simulink model "five_bar_model_with_gravity"  (R2018a)
settings: Solver=ode4  StartTime=0.0  StopTime=10  FixedStep=0.0001  RelTol=1e-3
values from neighbouring files (symbols this model uses):
  g = 9.80665    [ddyn5.m]    (also in idyn5.m = -9.80665; test_dynamics.m = -9.80665; test_model.m)
  q = [NaN; NaN; NaN; NaN; NaN]    [fkine5.m]    (also in ikine5.m = [q11;q12;q13;q21;q22])
  qa = [q11;q21]    [ikine5.m]    (also in model_parameters_v_1.m = ones(length(q_(1,:)),1) * 50; test_model.m = [q(1,:);q(4,:)])
  qda = Jinv * t0r    [ifirstkine5.m]    (also in test_model.m = [0.5; 0.5])
  t0r = J * qda    [ffirstkine5.m]    (also in test_dynamics.m = [0;0]; test_kinematics.m = [1;1]; test_model.m = p)
  t0rd = (J * qdda+ at)    [fsecondkine5.m]    (also in test_dynamics.m = [0;0]; test_kinematics.m = [-1;1]; test_model.m = p)
  x0 = p(1,1)    [model_parameters_v_1.m]    (also in test_model.m)
  y0 = p(2,1)    [model_parameters_v_1.m]    (also in test_model.m = p(1,2))
undefined symbols (not defined in the file or in its folder): X, Y, Z
libraries: sm_lib x25, nesl_utility x9, simulink x7, fl_lib x2
(part 2 of 2)

== matlab function five_bar_model_with_gravity/inverse first kinematics ==
  data: t0r input; qd output; p input double size=2; q input; qda output; qdu output; Ar output; B output; J output; Jinv output; Jt output; Jta output; Jtd output; Psit output
function [qd,qda,qdu,Ar,B,J,Jinv,Jt,Jta,Jtd,Psit] = ifirstkine5(t0r,p,q)
% This function implement the firs-order inverse kinematics model of a five bar robot
% @param t0r: twist end-effector vector 2X1
% @param p: end-effector coordinate vector 2X1
% @param q: joint positions vector 5x1
% @return qd: velocity joints vector 5x1
% @return qda: active velocity joints vector 2X1
% @return qdu: underactuated velocity joints vector 3X1
% @return Ar: matrix 2x2 relates the n dof independent coordinates of the platform twist 0 t r to the actuated joints q̇ a
% @return B: matrix 2x2 for computation of the dynamic model of the PKM
% @return J: kinematic Jacobian matrix of the PKM
% @return Jinv: inverse kinematic Jacobian matrix of the PKM
% @return Jt: crucial for computation of the dynamic model of the PKM.
% @return Jta: crucial for computation of the dynamic model of the PKM.
% @return Jtd: crucial for computation of the dynamic model of the PKM.
% @return Psit: matrix 2X6

    l = 0.205;
    d1 = [-0.125, l, l];
    d2 = [0.125, l, l];
    q1 = q(1:3);
    q2 = q(4:5);
    Phi = sum(q1);
    x = p(1);
    y = p(2);

    B = [ -d1(2)*sin(q1(2)), 0;
          0, -d2(2)*sin(q2(2))];


    Ar = [cos(q1(1) + q1(2)), sin(q1(1) + q1(2));
          cos(q2(1) + q2(2)), sin(q2(1) + q2(2))];
    % forward model
    J = -Ar \ B;
    % t0r = J * qda;
    % t0r =[ -(d1(2)*qd11*sin(q2(1) + q2(2))*sin(q1(2)) - ...
    %                 d2(2)*qd21*sin(q1(1) + q1(2))*sin(q2(2)))/sin(q1(1) + q1(2) - q2(1) - q2(2));
    %         (d1(2)*qd11*cos(q2(1) + q2(2))*sin(q1(2)) - ...
    %                 d2(2)*qd21*cos(q1(1) + q1(2))*sin(q2(2)))/sin(q1(1) + q1(2) - q2(1) - q2(2))];

    Jinv = -B \ Ar;
    qda = Jinv * t0r;
    % qda = [(xd*cos(q1(1) + q1(2)) + yd*sin(q1(1) + q1(2)))/(d1(2)*sin(q1(2)));
    %        (xd*cos(q2(1) + q2(2)) + yd*sin(q2(1) + q2(2)))/(d2(2)*sin(q2(2)))];


    ay = cos(Phi)^2 / (x - d2(2)*cos(q2(1)) - d2(1));
    ax = - ((y-d2(2)*sin(q2(1)))*cos(Phi)^2) / (x - d2(2)*cos(q2(1)) - d2(1))^2;
    aq = -(d2(2) * ((x-d2(1))*cos(q2(1))+y*sin(q2(1))-d2(2))*cos(Phi)^2) / (x - d2(2)*cos(q2(1)) - d2(1))^2;

    Psit = [1                     0
            0                     1
            0                     0
            0                     0
            0                     0
            (ax+aq*Jinv(2,1)) (ay+aq*Jinv(2,2))];

    Jt = [-sin(q1(1) + q1(2)),cos(q1(1) + q1(2));
            (ax + aq*Jinv(2,1)), (ay + aq*Jinv(2,2));
            -sin(q2(1) + q2(2)),cos(q2(1) + q2(2))];


    Jta = [ d1(3) + d1(2)*cos(q1(2)), 0;
            1,                0;
            0,      d2(3) + d2(2)*cos(q2(2))];

    Jtd = [ d1(3), 0,   0;
            1,   1,   0;
            0,   0, d2(3)];

    qdu = Jtd\(Jt * t0r - Jta * qda); 
    qd = [qda(1);qdu(1);qdu(2);qda(2);qdu(3)];

== matlab function five_bar_model_with_gravity/inverse secod kinematics ==
  data: t0rd input; qdd output; t0r input; p input double size=2; q input; qd input; Ar input; B input; Jinv input; Jt input; Jta input; Jtd input; Psit input; qdda output double size=2; qddu output; Psit1 output; Psit2 output; atp output; ad output
function [qdd,qdda,qddu,Psit1,Psit2,atp,ad] = isecondkine5(t0rd,t0r,p,q,qd,Ar,B,Jinv,Jt,Jta,Jtd,Psit)
% This function implement the second-order inverse kinematics model of a five bar robot
% @param t0rd: derivate twist end-effector vector 2X1
% @param t0r: twist end-effector vector 2X1
% @param p: end-effector coordinate vector 2X1
% @param q: joint positions vector 5x1
% @param qd: velocity joints vector 5x1
% @param Ar: matrix 2x2 for computation of the dynamic model of the PKM
% @param B: matrix 2x2 for computation of the dynamic model of the PKM
% @param Jinv: inverse kinematic Jacobian matrix of the PKM
% @param Jt: crucial for computation of the dynamic model of the PKM.
% @param Jta: crucial for computation of the dynamic model of the PKM.
% @param Jtd: crucial for computation of the dynamic model of the PKM.
% @return qdd: acceleration joint vector 5x1
% @return qdda: active acceleration joints vector 2X1
% @return qddu: underactuated acceleration joints vector 3X1
% @return Psit1: matrix 2x6
% @return Psit2: matrix 1x6
% @return atp: acceleration using for dynamics
% @return ad: acceleration using for dynamics

    l = 0.205;
    d1 = [-0.125, l, l];
    d2 = [0.125, l, l];
    q1 = q(1:3);
    q2 = q(4:5);
    qd1 = qd(1:3);
    qd2 = qd(4:5);
    Phi = sum(q1);
    Phid = sum(qd1);
    x = p(1);
    y = p(2);
    xd = t0r(1);
    yd = t0r(2);

    wr1 = [cos(q1(1)+q1(2)); sin(q1(1)+q1(2)); 0; 0; 0; 0];
    wr2 = [cos(q2(1)+q2(2)); sin(q2(1)+q2(2)); 0; 0; 0; 0];

    b01a_ = [-d1(2)*qd1(1)*cos(q1(1)) - d1(3)*cos(q1(1)+q1(2))*(qd1(1)+qd1(2));
             -d1(2)*qd1(1)*sin(q1(1)) - d1(3)*sin(q1(1)+q1(2))*(qd1(1)+qd1(2));
             zeros(4,1)];
    b01b_ = [-d1(3)*cos(q1(1)+q1(2));
             -d1(3)*sin(q1(1)+q1(2));
             zeros(4,1)];
    b0p1 = b01a_ * qd1(1) + b01b_ * qd1(2)*(qd1(1)+qd1(2));

    b02a_ = [-d2(2)*qd2(1)*cos(q2(1)) - d2(3)*cos(q2(1)+q2(2))*(qd2(1)+qd2(2));
             -d2(2)*qd2(1)*sin(q2(1)) - d2(3)*sin(q2(1)+q2(2))*(qd2(1)+qd2(2));
             zeros(4,1)];
    b02b_ = [-d2(3)*cos(q2(1)+q2(2));
             -d2(3)*sin(q2(1)+q2(2));
             zeros(4,1)];
    b0p2 = b02a_ * qd2(1) + b02b_ * qd2(2)*(qd2(1)+qd2(2));

    b0p = [(wr1'*b0p1); (wr2'*b0p2)];

    aqq = -B \ b0p;
    qdda = (Jinv * t0rd - aqq);

    % Aceleracion pasiva

    ayd = (Phid*sin(2*Phi))/(d2(1) - x + d2(2)*cos(q2(1))) - (cos(Phi)^2*(xd + d2(2)*qd2(1)*sin(q2(1))))/(d2(1) - x + d2(2)*cos(q2(1)))^2;

    axd = (Phid*sin(2*Phi)*(y - d2(2)*sin(q2(1))))/(d2(1) - x + d2(2)*cos(q2(1)))^2 ...
        - (cos(Phi)^2*(yd - d2(2)*qd2(1)*cos(q2(1))))/(d2(1) - x + d2(2)*cos(q2(1)))^2 ...
        - (2*cos(Phi)^2*(xd + d2(2)*qd2(1)*sin(q2(1)))*(y - d2(2)*sin(q2(1))))/(d2(1) - x + d2(2)*cos(q2(1)))^3;

    aqd = (2*d2(2)*cos(Phi)^2*(xd + d2(2)*qd2(1)*sin(q2(1)))*(d2(2) - sin(q2(1))*y + cos(q2(1))*(d2(1) - x)))...
        /(d2(1) - x + d2(2)*cos(q2(1)))^3 ...
        - (d2(2)*cos(Phi)^2*(xd*cos(q2(1)) + yd*sin(q2(1)) + qd2(1)*cos(q2(1))*y + qd2(1)*sin(q2(1))*(d2(1) - x)))...
        /(d2(1) - x + d2(2)*cos(q2(1)))^2 ...
        - (2*Phid*d2(2)*cos(Phi)*sin(Phi)*(d2(2) - sin(q2(1))*y + cos(q2(1))*(d2(1) - x)))...
        /(d2(1) - x + d2(2)*cos(q2(1)))^2;

    j21_invd = -(sin(q2(1) + q2(2))*(qd2(1) + qd2(2)))/(d2(2)*sin(q2(2))) ...
               -(qd2(2)*cos(q2(1) + q2(2))*cos(q2(2)))/(d2(2)*sin(q2(2))^2);

    j22_invd = -(qd2(2)*sin(q2(1) + q2(2))*cos(q2(2)))/(d2(2)*sin(q2(2))^2) ...
               +(cos(q2(1) + q2(2))*(qd2(1) + qd2(2)))/(d2(2)*sin(q2(2)));

    aq = -(d2(2) * ((x-d2(1))*cos(q2(1))+y*sin(q2(1))-d2(2))*cos(Phi)^2) / (x - d2(2)*cos(q2(1)) - d2(1))^2;

    psitd1 = axd + aqd*Jinv(2,1)+ aq*j21_invd;
    psitd2 = ayd + aqd*Jinv(2,2)+ aq*j22_invd;

    Psidt = [0 0; 0 0; 0 0; 0 0; 0 0; psitd1 psitd2];

    Psit1 = [-sin(q1(1)+q1(2)) cos(q1(1)+q1(2)) 0 0 0 0
             0                 0                0 0 0 1];
    Psit2 = [-sin(q2(1)+q2(2)) cos(q2(1)+q2(2)) 0 0 0 0];

    dc1 = Psit1 * (eye(6)* Psidt * t0r - b0p1);
    dc2 = Psit2 * (eye(6)* Psidt * t0r - b0p2);
    dc = [dc1;
          dc2];

    qddu =  Jtd\(Jt*t0rd - Jta*qdda + dc);

    qdd = [qdda(1);qddu(1);qddu(2);qdda(2);qddu(3)];

    at = -Ar \ b0p;
    atp = Psit * at + Psidt * t0r;% using for dynamics
    ad = Jtd \ (dc + Jt*at); % For dynamics

== matlab function five_bar_model_with_gravity/forward kinematics ==
  data: qa_act input double size=2; p_act output double size=2; q_act output double size=5; p_ant input double size=2; q_ant input double size=5; flag_velocity output; t0r input; t0rd input; dt input; assembly1_ input boolean
function [p_act, q_act, flag_velocity]  = fkine5(qa_act, p_ant, q_ant, t0r, t0rd, dt, assembly1_)
% This function implement the forward kinematic model of a five bar robot
% @parm q: joint positions vector 5x1
% @return p: p end-effector coordinate vector 2X1
    l = 0.205;
    d1 = [-0.125, l, l];
    d2 = [0.125, l, l];
    q1 = qa_act(1);
    q2 = qa_act(2);
    

    A12 = [d1(2)*cos(q1(1))+d1(1); d1(2)*sin(q1(1))];
    A22 = [d2(2)*cos(q2(1))+d2(1); d2(2)*sin(q2(1))];
    s = sqrt(sum((A22-A12).^2));
    if s <= 2*l 
        flag_velocity=0;

        if assembly1_
            a1 = - 2*d1(1) - 2*d1(2)*cos(q1(1));
            a2 = - 2*d2(1) - 2*d2(2)*cos(q2(1));
            b1 = - 2*sin(q1(1))*d1(2);
            b2 = - 2*sin(q2(1))*d2(2);
            c1 = d1(1)^2 + 2*cos(q1(1))*d1(1)*d1(2) + d1(2)^2 - d1(3)^2;
            c2 = d2(1)^2 + 2*cos(q2(1))*d2(1)*d2(2) + d2(2)^2 - d2(3)^2;

            if b1 ~= b2
                a = a2 - a1;
                b = b2 - b1;
                c = c2 - c1;
                e1 = - a / b;
                e2 = - c / b;
                f1 = 1 + e1^2;
                f2 = 2 * e1 * e2 + a1 + b1 * e1;
                f3 = e2^2 + b1 * e2 + c1;

                x = (-f2 - sqrt(f2^2 - 4 * f1 * f3)) / (2 * f1);
                y = e1 * x + e2;

                A13=[x-A12(1);y-A12(2)];
                A23=[x-A22(1);y-A22(2)];
                if  A13(1)*A23(2)-A23(1)*A13(2) <= 0
                    x = (-f2 + sqrt(f2^2 - 4 * f1 * f3)) / (2 * f1);
                    y = e1 * x + e2;
                end
            else
                x = - (c2 - c1) / (a2 - a1);
                y = (-b1 + (b1^2 - 4 * (x^2 + a1 * x + c1))^(1/2)) / 2;

                A13=[x-A12(1);y-A12(2)];
                A23=[x-A22(1);y-A22(2)];
                if  A13(1)*A23(2)-A23(1)*A13(2) <= 0
                    y = (-b1 - (b1^2 - 4 * (x^2 + a1 * x + c1))^(1/2)) / 2;
                end
            end

            % for q12 and q22 from a12/a11 and a22/a21
            q12 = atan2(y-d1(2)*sin(q1(1)), x-d1(1)-d1(2)*cos(q1(1))) - q1(1);
            q22 = atan2(y-d2(2)*sin(q2(1)), x-d2(1)-d2(2)*cos(q2(1))) - q2(1);
            q13 = q2(1) + q22 - q1(1) - q12;
            q_act = [q1(1); q12; q13; q2(1); q22];
            p_act = [x;y];
            
            dist013 = sqrt((p_act(1)-d1(1))^2+p_act(2)^2);
            dist023 = sqrt((p_act(1)-d2(1))^2+p_act(2)^2);
            if dist013 > 2*l || dist023 > 2*l || (p_act-p_ant)'*(p_act-p_ant)>0.01
%                 disp('Warning: dist>2*l');
% %                 change_ass = true;
%                 flag_velocity = 1;
%                 p_act = p_ant;%+ t0rd * dt^2 / 2 + t0r * dt;
% %                 q_act = q_ant;
%             else
%                 flag_velocity=0;
%             end
                     
                disp('assembly 2');
                a1 = - 2*d1(1) - 2*d1(2)*cos(q1(1));
                a2 = - 2*d2(1) - 2*d2(2)*cos(q2(1));
                b1 = - 2*sin(q1(1))*d1(2);
                b2 = - 2*sin(q2(1))*d2(2);
                c1 = d1(1)^2 + 2*cos(q1(1))*d1(1)*d1(2) + d1(2)^2 - d1(3)^2;
                c2 = d2(1)^2 + 2*cos(q2(1))*d2(1)*d2(2) + d2(2)^2 - d2(3)^2;

                if b1 ~= b2
                    a = a2 - a1;
                    b = b2 - b1;
                    c = c2 - c1;
                    e1 = - a / b;
                    e2 = - c / b;
                    f1 = 1 + e1^2;
                    f2 = 2 * e1 * e2 + a1 + b1 * e1;
                    f3 = e2^2 + b1 * e2 + c1;

                    x = (-f2 - sqrt(f2^2 - 4 * f1 * f3)) / (2 * f1);
                    y = e1 * x + e2;

                    A13=[x-A12(1);y-A12(2)];
                    A23=[x-A22(1);y-A22(2)];
                    if  A13(1)*A23(2)-A23(1)*A13(2) >= 0
                        x = (-f2 + sqrt(f2^2 - 4 * f1 * f3)) / (2 * f1);
                        y = e1 * x + e2;
                    end
                else
                    x = - (c2 - c1) / (a2 - a1);
                    y = (-b1 + (b1^2 - 4 * (x^2 + a1 * x + c1))^(1/2)) / 2;

                    A13=[x-A12(1);y-A12(2)];
                    A23=[x-A22(1);y-A22(2)];
                    if  A13(1)*A23(2)-A23(1)*A13(2) >= 0
                        y = (-b1 - (b1^2 - 4 * (x^2 + a1 * x + c1))^(1/2)) / 2;
                    end
                end

                % for q12 and q22 from a12/a11 and a22/a21
                q12 = atan2(y-d1(2)*sin(q1(1)), x-d1(1)-d1(2)*cos(q1(1))) - q1(1);
                q22 = atan2(y-d2(2)*sin(q2(1)), x-d2(1)-d2(2)*cos(q2(1))) - q2(1);
                q13 = q2(1) + q22 - q1(1) - q12;
                q_act = [q1(1); q12; q13; q2(1); q22];
                p_act = [x;y];
            
            dist013 = sqrt((p_act(1)-d1(1))^2+p_act(2)^2);
            dist023 = sqrt((p_act(1)-d2(1))^2+p_act(2)^2);
            if dist013 > 2*l || dist023 > 2*l
                disp('Warning: dist>2*l');
%                 change_ass = true;
                flag_velocity = 1;
                p_act = p_ant;%+ t0rd * dt^2 / 2 + t0r * dt;
                q_act = q_ant;
            end
%             else
%                 flag_velocity=0;
%             end
            end
        else
            p_act = p_ant;
            q_act = q_ant;
        end
%         change_ass = false;

    else       
        q_ = zeros(5,4);
        disp('Warning: s>2*l');
%         change_ass = true;
        flag_velocity = 0;
        p_act = p_ant + t0rd * dt^2 / 2 + t0r * dt;
%         q_act = q_ant;
        % find  previous working mode
        A11_12_ant = [d1(2)*cos(q_ant(1))+d1(1); d1(2)*sin(q_ant(1))];
        A21_22_ant = [d2(2)*cos(q_ant(4))+d2(1); d2(2)*sin(q_ant(4))];
        A12_13_ant = p_ant - A11_12_ant;
        A22_23_ant = p_ant - A21_22_ant;
        A12_11_ant = [d1(1); 0] - A11_12_ant;
        A22_21_ant = [d2(1); 0] - A21_22_ant;
        work_mode1 = sign(A12_13_ant(1) * A12_11_ant(2) ...
                        - A12_13_ant(2) * A12_11_ant(1));
        work_mode2 = sign(A22_23_ant(1) * A22_21_ant(2) ...
                        - A22_23_ant(2) * A22_21_ant(1));
        % inverse kinematics
            dist013 = sqrt((p_act(1)-d1(1))^2+p_act(2)^2);
            dist023 = sqrt((p_act(1)-d2(1))^2+p_act(2)^2);
            if dist013 <= 2*l && dist023 <= 2*l
                disp('Information: inverse kinematics calculation');
                x = p_act(1);
                y = p_act(2);
                q11 = -2*atan((((d1(1)^2 - 2*d1(1)*x - d1(2)^2 + 2*d1(2)*d1(3) - d1(3)^2 + x^2 + y^2)*(- d1(1)^2 + 2*d1(1)*x + d1(2)^2 + 2*d1(2)*d1(3) + d1(3)^2 - x^2 - y^2))^(1/2) - 2*d1(2)*y)/(d1(1)^2 - 2*d1(1)*d1(2) - 2*d1(1)*x + d1(2)^2 + 2*d1(2)*x - d1(3)^2 + x^2 + y^2));
                if ~isreal(q11)
                    q_(:,1) = [NaN, NaN, NaN, NaN, NaN]';
                    q_(:,2) = [NaN, NaN, NaN, NaN, NaN]';
                else
                    q21 = -2*atan((((d2(1)^2 - 2*d2(1)*x - d2(2)^2 + 2*d2(2)*d2(3) - d2(3)^2 + x^2 + y^2)*(- d2(1)^2 + 2*d2(1)*x + d2(2)^2 + 2*d2(2)*d2(3) + d2(3)^2 - x^2 - y^2))^(1/2) - 2*d2(2)*y)/(d2(1)^2 - 2*d2(1)*d2(2) - 2*d2(1)*x + d2(2)^2 + 2*d2(2)*x - d2(3)^2 + x^2 + y^2));
                    if ~isreal(q21)
                        q_(:,1) = [NaN, NaN, NaN, NaN, NaN]';
                    else
%                         A12 = [d1(2)*cos(q11)+d1(1); d1(2)*sin(q11)];
%                         A22 = [d2(2)*cos(q21)+d2(1); d2(2)*sin(q21)];
%                         A13=[A12(1)-x;A12(2)-y];
%                         A23=[A22(1)-x;A22(2)-y];
%                         if  A13(1)*A23(2)-A23(1)*A13(2) <= 0
%                             q_(:,1) = [NaN, NaN, NaN, NaN, NaN]';
%                         else
                            q12 = - q11 + atan2(y - d1(2)*sin(q11), x - d1(1) - d1(2)*cos(q11));
                            q22 = - q21 + atan2(y - d2(2)*sin(q21), x - d2(1) - d2(2)*cos(q21));
                            q13 = q21 - q12 - q11 + q22;
                            q_(:,1) = [q11, q12, q13, q21, q22]';
%                         end
                    end
                    q21 = 2*atan((((d2(1)^2 - 2*d2(1)*x - d2(2)^2 + 2*d2(2)*d2(3) - d2(3)^2 + x^2 + y^2)*(- d2(1)^2 + 2*d2(1)*x + d2(2)^2 + 2*d2(2)*d2(3) + d2(3)^2 - x^2 - y^2))^(1/2) + 2*d2(2)*y)/(d2(1)^2 - 2*d2(1)*d2(2) - 2*d2(1)*x + d2(2)^2 + 2*d2(2)*x - d2(3)^2 + x^2 + y^2));
                    if ~isreal(q21)
                        q_(:,2) = [NaN, NaN, NaN, NaN, NaN]';
                    else
%                         A12 = [d1(2)*cos(q11)+d1(1); d1(2)*sin(q11)];
%                         A22 = [d2(2)*cos(q21)+d2(1); d2(2)*sin(q21)];
%                         A13=[A12(1)-x;A12(2)-y];
%                         A23=[A22(1)-x;A22(2)-y];
%                         if  A13(1)*A23(2)-A23(1)*A13(2) <= 0
%                             q_(:,2) = [NaN, NaN, NaN, NaN, NaN]';
%                         else
                            q12 = - q11 + atan2(y - d1(2)*sin(q11), x - d1(1) - d1(2)*cos(q11));
                            q22 = - q21 + atan2(y - d2(2)*sin(q21), x - d2(1) - d2(2)*cos(q21));
                            q13 = q21 - q12 - q11 + q22;
                            q_(:,2) = [q11, q12, q13, q21, q22]';
%                         end
                    end
                end

                q11 = 2*atan((((d1(1)^2 - 2*d1(1)*x - d1(2)^2 + 2*d1(2)*d1(3) - d1(3)^2 + x^2 + y^2)*(- d1(1)^2 + 2*d1(1)*x + d1(2)^2 + 2*d1(2)*d1(3) + d1(3)^2 - x^2 - y^2))^(1/2) + 2*d1(2)*y)/(d1(1)^2 - 2*d1(1)*d1(2) - 2*d1(1)*x + d1(2)^2 + 2*d1(2)*x - d1(3)^2 + x^2 + y^2));
                if ~isreal(q11)
                    q_(:,3) = [NaN, NaN, NaN, NaN, NaN]';
                    q_(:,4) = [NaN, NaN, NaN, NaN, NaN]';
                else
                    q21 = -2*atan((((d2(1)^2 - 2*d2(1)*x - d2(2)^2 + 2*d2(2)*d2(3) - d2(3)^2 + x^2 + y^2)*(- d2(1)^2 + 2*d2(1)*x + d2(2)^2 + 2*d2(2)*d2(3) + d2(3)^2 - x^2 - y^2))^(1/2) - 2*d2(2)*y)/(d2(1)^2 - 2*d2(1)*d2(2) - 2*d2(1)*x + d2(2)^2 + 2*d2(2)*x - d2(3)^2 + x^2 + y^2));
                    if ~isreal(q21)
                        q_(:,3) = [NaN, NaN, NaN, NaN, NaN]';
                    else
%                         A12 = [d1(2)*cos(q11)+d1(1); d1(2)*sin(q11)];
%                         A22 = [d2(2)*cos(q21)+d2(1); d2(2)*sin(q21)];
%                         A13=[A12(1)-x;A12(2)-y];
%                         A23=[A22(1)-x;A22(2)-y];
%                         if  A13(1)*A23(2)-A23(1)*A13(2) <= 0
%                             q_(:,3) = [NaN, NaN, NaN, NaN, NaN]';
%                         else
                            q12 = - q11 + atan2(y - d1(2)*sin(q11), x - d1(1) - d1(2)*cos(q11));
                            q22 = - q21 + atan2(y - d2(2)*sin(q21), x - d2(1) - d2(2)*cos(q21));
                            q13 = q21 - q12 - q11 + q22;
                            q_(:,3) = [q11, q12, q13, q21, q22]';
%                         end
                    end
                    q21 = 2*atan((((d2(1)^2 - 2*d2(1)*x - d2(2)^2 + 2*d2(2)*d2(3) - d2(3)^2 + x^2 + y^2)*(- d2(1)^2 + 2*d2(1)*x + d2(2)^2 + 2*d2(2)*d2(3) + d2(3)^2 - x^2 - y^2))^(1/2) + 2*d2(2)*y)/(d2(1)^2 - 2*d2(1)*d2(2) - 2*d2(1)*x + d2(2)^2 + 2*d2(2)*x - d2(3)^2 + x^2 + y^2));
                    if ~isreal(q21)
                        q_(:,4) = [NaN, NaN, NaN, NaN, NaN]';
                    else
%                         A12 = [d1(2)*cos(q11)+d1(1); d1(2)*sin(q11)];
%                         A22 = [d2(2)*cos(q21)+d2(1); d2(2)*sin(q21)];
%                         A13=[A12(1)-x;A12(2)-y];
%                         A23=[A22(1)-x;A22(2)-y];
%                         if  A13(1)*A23(2)-A23(1)*A13(2) <= 0
%                             q_(:,4) = [NaN, NaN, NaN, NaN, NaN]';
%                         else
                            q12 = - q11 + atan2(y - d1(2)*sin(q11), x - d1(1) - d1(2)*cos(q11));
                            q22 = - q21 + atan2(y - d2(2)*sin(q21), x - d2(1) - d2(2)*cos(q21));
                            q13 = q21 - q12 - q11 + q22;
                            q_(:,4) = [q11, q12, q13, q21, q22]';
%                         end
                    end
                end 
                if ~isnan(q_(1,1)) || ~isnan(q_(1,2)) || ~isnan(q_(1,3)) ...
                        || ~isnan(q_(1,4))
                    index = 1;
                    for i=1:4 
                        if isnan(q_(1,i))
                            continue;
                        else
                            % The courrent working mode must be the same
                            % that the previous
                            A11_12 = [d1(2)*cos(q_(1,i))+d1(1); d1(2)*sin(q_(1,i))];
                            A21_22 = [d2(2)*cos(q_(4,i))+d2(1); d2(2)*sin(q_(4,i))];
                            A12_13 = p_act - A11_12;
                            A22_23 = p_act - A21_22;
                            A12_11 = [d1(1); 0] - A11_12;
                            A22_21 = [d2(1); 0] - A21_22;
                            work_mode1_act = sign(A12_13(1) * A12_11(2) - A12_13(2) * A12_11(1));
                            work_mode2_act = sign(A22_23(1) * A22_21(2) - A22_23(2) * A22_21(1));

                            if isequal(work_mode1, work_mode1_act) && ...
                                    isequal(work_mode2, work_mode2_act)
                                index = i;
                                break;
                            else
                                continue;
                            end
                        end
                    end
                
%                     q_ant
                    
                    q_act = q_(:, index);
                    index
                    suma = sum(angdiff(q_,q_ant*ones(1,4)).^2)
                    aux = find(suma==min(suma))
                    q_act = q_(:, aux(1));
%                     pause();
                else
                    flag_velocity = 1;
                    q_act = q_ant;
                end
            else
                flag_velocity = 1;
                q_act = q_ant;
                pause();
            end
            

%         x = p(1);
%         y = p(2);
%         q1(1) = q_ant(1);
%         q2(1) = q_ant(2);
%         q12 = atan2(y-d1(2)*sin(q1(1)), x-d1(1)-d1(2)*cos(q1(1))) - q1(1);
%         q22 = atan2(y-d2(2)*sin(q2(1)), x-d2(1)-d2(2)*cos(q2(1))) - q2(1);
%         q13 = q2(1) + q22 - q1(1) - q12;
%         q_ = [q1(1); q12; q13; q2(1); q22];
      
    end

== matlab function five_bar_model_with_gravity/second forward kinematics ==
  data: qdda input; t0rd output double size=2; qd input; q input; Ar input; J input
function t0rd  = fsecondkine5(qdda,qd,q,Ar,J)
% This function implement the second-order forward kinematics model of a five bar robot
% @param qdda: active acceleration joints vector 2X1
% @param qd: velocity joints vector 5x1
% @param q: joint positions vector 5x1
% @param Ar: matrix 2x2 for computation of the dynamic model of the PKM
% @param J: kinematic Jacobian matrix of the PKM
% @return t0rd: derivate twist end-effector vector 2X1
    l = 0.205;
    d1 = [-0.125, l, l];
    d2 = [0.125, l, l];
    q1 = q(1:3);
    q2 = q(4:5);
    qd1 = qd(1:3);
    qd2 = qd(4:5);

    wr1 = [cos(q1(1)+q1(2)); sin(q1(1)+q1(2)); 0; 0; 0; 0];
    wr2 = [cos(q2(1)+q2(2)); sin(q2(1)+q2(2)); 0; 0; 0; 0];

    b01a_ = [-d1(2)*qd1(1)*cos(q1(1)) - d1(3)*cos(q1(1)+q1(2))*(qd1(1)+qd1(2));
             -d1(2)*qd1(1)*sin(q1(1)) - d1(3)*sin(q1(1)+q1(2))*(qd1(1)+qd1(2));
             zeros(4,1)];
    b01b_ = [-d1(3)*cos(q1(1)+q1(2));
             -d1(3)*sin(q1(1)+q1(2));
             zeros(4,1)];
    b0p1 = b01a_ * qd1(1) + b01b_ * qd1(2)*(qd1(1)+qd1(2));

    b02a_ = [-d2(2)*qd2(1)*cos(q2(1)) - d2(3)*cos(q2(1)+q2(2))*(qd2(1)+qd2(2));
             -d2(2)*qd2(1)*sin(q2(1)) - d2(3)*sin(q2(1)+q2(2))*(qd2(1)+qd2(2));
             zeros(4,1)];
    b02b_ = [-d2(3)*cos(q2(1)+q2(2));
             -d2(3)*sin(q2(1)+q2(2));
             zeros(4,1)];
    b0p2 = b02a_ * qd2(1) + b02b_ * qd2(2)*(qd2(1)+qd2(2));

    b0p = [(wr1'*b0p1); (wr2'*b0p2)];

    at = Ar\b0p;
    t0rd = (J * qdda+ at);

== matlab function five_bar_model_with_gravity/MATLAB Function ==
  data: q input; assembly_mode_ input; assembly_mode output
function assembly_mode = fcn(q,assembly_mode_)
l = 0.205;
d1 = [-0.125, l, l];
d2 = [0.125, l, l];
q11 = q(1);
q21 = q(4);
A12 = [d1(2)*cos(q11)+d1(1); d1(2)*sin(q11)];
A22 = [d2(2)*cos(q21)+d2(1); d2(2)*sin(q21)];
s = sqrt(sum((A22-A12).^2));
if abs(q(1) + q(2) -q(4) - q(5)) < 0.1 ...
        ||  abs(abs(q(1) + q(2) -q(4) - q(5)) - pi) < 0.1 || s>(2*l-0.01)
    if assembly_mode_ == 1
        assembly_mode = -1;
    else
        assembly_mode = 1;
    end
else
    if assembly_mode_ == 1
        assembly_mode = 1;
    else
        assembly_mode = -1;
    end
end

== matlab function five_bar_model_with_gravity/fkniematics simple ==
  data: qa input; q output size=5; assembly_mode input; p output; p_ant input; q_ant input; flag_vel output size=1
function [q, p, flag_vel] = fkinematics(qa, assembly_mode,p_ant,q_ant)
% Assembly_mode 1+ o 1-
l = 0.205;
d1 = [-0.125, l, l];
d2 = [0.125, l, l];
q11 = qa(1);
q21 = qa(2);
A12 = [d1(2)*cos(q11)+d1(1); d1(2)*sin(q11)];
A22 = [d2(2)*cos(q21)+d2(1); d2(2)*sin(q21)];
s = sqrt(sum((A22-A12).^2));
if s <= 2*l    
    a1 = - 2*d1(1) - 2*d1(2)*cos(q11);
    a2 = - 2*d2(1) - 2*d2(2)*cos(q21);
    b1 = - 2*sin(q11)*d1(2);
    b2 = - 2*sin(q21)*d2(2);
    c1 = d1(1)^2 + 2*cos(q11)*d1(1)*d1(2) + d1(2)^2 - d1(3)^2;
    c2 = d2(1)^2 + 2*cos(q21)*d2(1)*d2(2) + d2(2)^2 - d2(3)^2;
    if b1 ~= b2
        a = a2 - a1;
        b = b2 - b1;
        c = c2 - c1;
        e1 = - a / b;
        e2 = - c / b;
        f1 = 1 + e1^2;
        f2 = 2 * e1 * e2 + a1 + b1 * e1;
        f3 = e2^2 + b1 * e2 + c1;

        x = (-f2 - sqrt(f2^2 - 4 * f1 * f3)) / (2 * f1);
        y = e1 * x + e2;

        A13=[x-A12(1);y-A12(2)];
        A23=[x-A22(1);y-A22(2)];
        if assembly_mode == 1 && A13(1)*A23(2)-A23(1)*A13(2) < 0  
            x = (-f2 + sqrt(f2^2 - 4 * f1 * f3)) / (2 * f1);
            y = e1 * x + e2;
        elseif assembly_mode == -1 && A13(1)*A23(2)-A23(1)*A13(2) > 0
            x = (-f2 + sqrt(f2^2 - 4 * f1 * f3)) / (2 * f1);
            y = e1 * x + e2;
        end
    else
        x = - (c2 - c1) / (a2 - a1);
        y = (-b1 + (b1^2 - 4 * (x^2 + a1 * x + c1))^(1/2)) / 2;

        A13=[x-A12(1);y-A12(2)];
        A23=[x-A22(1);y-A22(2)];
        if assembly_mode == 1 && A13(1)*A23(2)-A23(1)*A13(2) < 0
            y = (-b1 - (b1^2 - 4 * (x^2 + a1 * x + c1))^(1/2)) / 2;
        elseif assembly_mode == -1 && A13(1)*A23(2)-A23(1)*A13(2) > 0
            y = (-b1 - (b1^2 - 4 * (x^2 + a1 * x + c1))^(1/2)) / 2;
        end
    end
    % for q12 and q22 from a12/a11 and a22/a21
    q12 = atan2(y-d1(2)*sin(q11), x-d1(1)-d1(2)*cos(q11)) - q11;
    q22 = atan2(y-d2(2)*sin(q21), x-d2(1)-d2(2)*cos(q21)) - q21;
    q13 = q21 + q22 - q11 - q12;
    q = [q11; q12; q13; q21; q22];
    p = [x;y];
    flag_vel=0;
else
    disp('Out of work space');
%     assembly_mode = -assembly_mode_ant;
%     q = [NaN; NaN; NaN; NaN; NaN];
    q = q_ant;
    p = p_ant;%[NaN; NaN];
    flag_vel = 1;
%     y = p(2);
%     x = p(1);
%     q11 = q_ant(1) - sign(q_ant(1))*0.001;
%     q21 = q_ant(4) - sign(q_ant(4))*0.001;
%     q12 = atan2(y-d1(2)*sin(q11), x-d1(1)-d1(2)*cos(q11)) - q11;
%     q22 = atan2(y-d2(2)*sin(q21), x-d2(1)-d2(2)*cos(q21)) - q21;
%     q13 = q21 + q22 - q11 - q12;
%     q = [q11; q12; q13; q21; q22];
end
